simulink model "alinea5"  (R2017b)
settings: Solver=VariableStepAuto  StartTime=0.0  StopTime=10.0  MaxStep=0.01  RelTol=1e-3
settings Model: Creator=Rita Monteiro  LastModifiedBy=Rita Monteiro
settings DebuggingCC: AlgebraicLoopMsg=none

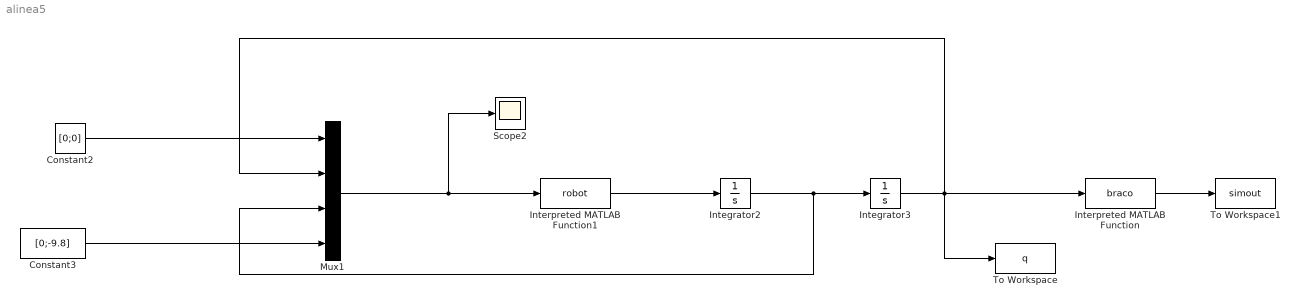
== system alinea5 ==
  Constant2 : Constant  Value=[0;0]  VectorParams1D=off
  Constant3 : Constant  Value=[0;-9.8]  VectorParams1D=off
  Integrator2 : Integrator  InitialCondition=[0;0]
  Integrator3 : Integrator  InitialCondition=[pi/2;pi/4]
  Interpreted MATLAB Function : MATLABFcn  MATLABFcn=braco  OutputDimensions=1
  Interpreted MATLAB Function1 : MATLABFcn  MATLABFcn=robot
  Mux1 : Mux
  Scope2 : Scope
  To Workspace : ToWorkspace  VariableName=q
  To Workspace1 : ToWorkspace  VariableName=simout  SampleTime=-1
  wires:
  Constant3/1 -> Mux1/4
  Constant2/1 -> Mux1/1
  Mux1/1 -> Scope2/1, Interpreted MATLAB Function1/1
  Interpreted MATLAB Function1/1 -> Integrator2/1
  Integrator3/1 -> To Workspace/1, Interpreted MATLAB Function/1, Mux1/2
  Integrator2/1 -> Mux1/3, Integrator3/1
  Interpreted MATLAB Function/1 -> To Workspace1/1
